simulink model "IO503nointerrupt"  (Simulink 7.3)
settings: Solver=FixedStepDiscrete  StartTime=0.0  StopTime=inf  RelTol=1e-3
InitFcn:
  | Ts = 0.1;
undefined symbols (not defined in the file): standard
libraries: speedgoatlib x5, xpclib x1, simulink x1
settings Model: Creator=dkuratli  LastModifiedBy=lab3  BufferReuse=off
settings DataIOCC: ReturnWorkspaceOutputs=off
settings OptimizationCC: BlockReduction=off  OptimizeBlockIOStorage=off  BufferReuse=off  ExpressionFolding=off  ExpressionDepthLimit=128  LocalBlockOutputs=off
settings DebuggingCC: UnderspecifiedInitializationDetection=Simplified  FcnCallInpInsideContextMsg=Enable All  StateNameClashWarn=none  StrictBusMsg=ErrorLevel1
settings HardwareCC: ProdIntDivRoundTo=Zero  ProdEndianess=LittleEndian  ProdHWDeviceType=Generic->32-bit x86 compatible
settings RTWCC: SystemTargetFile=xpctarget.tlc  TemplateMakefile=xpc_default_tmf  Description=Simulink Real-Time  RTWVerbose=off  ProcessScript=xpctarget_make_rtw_hook  RTWCompilerOptimization=On
settings CodeAppCC: CustomSymbolStrType=$N$R$M_T
settings xpcTargetCC: TargetFcnLib=ansi_tfl_table_tmw.mat  TargetFunctionLibrary=ANSI_C  ParMdlRefBuildCompliant=on  ConcurrentExecutionCompliant=on  CombineSignalStateStructs=off  GRTInterface=on  GenerateAllocFcn=off  xPCTaskExecutionProfile=off  xPCRL32EventNumber=5000  xPCLoadParamSetFile=off  xPCConcurrentTasks=off  xPCEnableSFAnimation=off

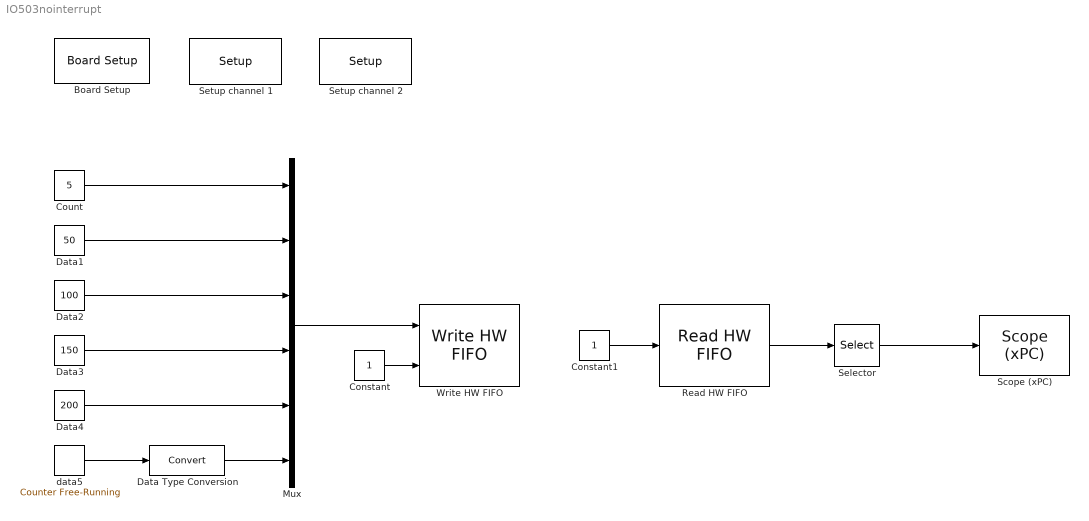
== system IO503nointerrupt ==
  Board Setup : speedgoatlib/IO503/Speedgoat IO503 Internal blocks/Board Setup  irqnum=10  slot=-1
  Constant : Constant  OutDataTypeStr=Inherit: Inherit via back propagation  SampleTime=Ts
  Constant1 : Constant  OutDataTypeStr=Inherit: Inherit via back propagation  SampleTime=Ts
  Count : Constant  Value=5  OutDataTypeStr=Inherit: Inherit via back propagation  SampleTime=Ts
  Data Type Conversion : DataTypeConversion
  Data1 : Constant  Value=50  OutDataTypeStr=Inherit: Inherit via back propagation  SampleTime=Ts
  Data2 : Constant  Value=100  OutDataTypeStr=Inherit: Inherit via back propagation  SampleTime=Ts
  Data3 : Constant  Value=150  OutDataTypeStr=Inherit: Inherit via back propagation  SampleTime=Ts
  Data4 : Constant  Value=200  OutDataTypeStr=Inherit: Inherit via back propagation  SampleTime=Ts
  Mux : Mux  Inputs=6
  Read HW FIFO : speedgoatlib/IO503/Speedgoat IO503 Internal blocks/Read HW FIFO  port=2  flush=on  slot=-1
  Scope (xPC) : xpclib/Misc./Scope (xPC)   scopeno=2  scopetype=Target  autostart=on  viewmode=Numerical  formatstr='%15.6f'  grid=on  ylimits=[0,0]  nosamples=3  noprepostsamples=0  interleave=1  triggermode=FreeRun  triggersignal=1  trigsignalfromport=off  triggerlevel=0.0  triggerslope=Either  triggerscope=1  triggersample=0  filename=data.dat  mode=Lazy  writesize=512  autorestart=off  dynamicfilemode=off  maxwritefilesize=512*1024^2
  Selector : Selector  InputPortWidth=65  Indices=[1:6]
  "Setup channel 1 " : speedgoatlib/IO503/Speedgoat IO503 Internal blocks/Setup  port=1  transceiver=RS232 (max 921.6kb/s)  standard=on  baudrate=115200  bauddivisor=1  mode8x=16x (standard)  prescale=off  width=8  nstop=1  parity=None  rlevel=1  ctsmode=none  xonoff=none  xon=17  xoff=19  rs485mode=off  rs485delay=0  slot=-1
  Setup channel 2 : speedgoatlib/IO503/Speedgoat IO503 Internal blocks/Setup  port=2  transceiver=RS232 (max 921.6kb/s)  standard=on  baudrate=115200  bauddivisor=1  mode8x=16x (standard)  prescale=off  width=8  nstop=1  parity=None  rlevel=1  ctsmode=none  xonoff=none  xon=17  xoff=19  rs485mode=off  rs485delay=0  slot=-1
  Write HW FIFO : speedgoatlib/IO503/Speedgoat IO503 Internal blocks/Write HW FIFO  port=1  slot=-1
  data5 : simulink/Sources/Counter Free-Running  NumBits=8  tsamp=Ts
  wires:
  Constant1/1 -> Read HW FIFO/1
  Constant/1 -> Write HW FIFO/2
  Count/1 -> Mux/1
  Data1/1 -> Mux/2
  data5/1 -> Data Type Conversion/1
  Data Type Conversion/1 -> Mux/6
  Mux/1 -> Write HW FIFO/1
  Data2/1 -> Mux/3
  Data3/1 -> Mux/4
  Data4/1 -> Mux/5
  Read HW FIFO/1 -> Selector/1
  Selector/1 -> Scope (xPC)/1
